simulink model "NavFilterTestHarness24"  (R2016b)
settings: Solver=FixedStepDiscrete  StartTime=startTime  StopTime=endTime  FixedStep=0.001  RelTol=1e-3  EnableMultiTasking=on
undefined symbols (not defined in the file): accel, ADSframe, ADStime, alignTime, angRate, ATTframe, CourseDeg, EAS2TAS, GndSpd, GPSframe, GPStime, Hgt, IMUframe, IMUtime, LatDeg, LngDeg, MagBiasX, MagBiasY, MagBiasZ, MAGframe, MAGtime, MagX, MagY, MagZ, msecHgtDelay, msecMagDelay, msecPosDelay, msecTasDelay, msecVelDelay, Pitch, Roll, Veas, VelD, Yaw
libraries: simulink x9, simulink_need_slupdate x2
(part 4 of 5)

== matlab function NavFilterTestHarness24/InertialNavFilter/Fuse True Airspeed Measurements ==
  data: states input; P input; FuseData input; VtasMea input; nextStates output; nextP output; innovation output; StatesAtMeasTime input; varInnov output; useAirspeed input
%#codegen
function [...
    nextStates, ... % state vector after fusion of measurements
    nextP, ... % state covariance matrix after fusion of corrections
    innovation, ... % True airspeed innovations (m/s)
    varInnov] ... % True airspeed innovation variance (m/s)^2
    = FuseAirspeed( ...
    states, ... % predicted states from the INS (q0, ... , q3, VelN,E,D, PosN,E,D, WindN,E, P0, camera roll pitch yaw misalignment)
    P, ... % predicted covariance
    FuseData, ... % Boolean to initiate fusion of airspeed measurements
    VtasMea, ... % true airspeed measurement (m/s)
    StatesAtMeasTime, ... % states at time of airspeed measurement
    useAirspeed) % Boolean to indicate that a airspeed sensor is being used

% define arrays used to calculate intermediate result in covariance
% update
KH  = single(zeros(24,24));
KHP = single(zeros(24,24));

% initialise innovation
innovation = single(0);

% initialise innovation variance vector (for data analysis only)
varInnov = single(0);

% Airspeed measurement error variance (m/s)^2.
R_TAS = single(2.0);

% Copy required states to local variable names
vn = single(StatesAtMeasTime(5));
ve = single(StatesAtMeasTime(6));
vd = single(StatesAtMeasTime(7));
vwn = single(StatesAtMeasTime(17));
vwe = single(StatesAtMeasTime(18));

% Calculate the airspeed prediction
VtasPred = sqrt((ve - vwe)^2 + (vn - vwn)^2 + vd^2);
% Need to check that it is flying before fusing airspeed data due to
if (useAirspeed && FuseData && (VtasPred > 1.0) && VtasMea > 8.0)
    % Sequential fusion of XYZ components
    
    % Calculate observation jacobians
    SH_TAS = single(zeros(3,1));
    SH_TAS(1) = 1/VtasPred;
    SH_TAS(2) = (SH_TAS(1)*(2*ve - 2*vwe))/2;
    SH_TAS(3) = (SH_TAS(1)*(2*vn - 2*vwn))/2;
    
    H_TAS = single(zeros(1,24));
    H_TAS(1,5) = SH_TAS(3);
    H_TAS(1,6) = SH_TAS(2);
    H_TAS(1,7) = vd*SH_TAS(1);
    H_TAS(1,17) = -SH_TAS(3);
    H_TAS(1,18) = -SH_TAS(2);
    
    SK_TAS = 1/(R_TAS + SH_TAS(3)*(P(5,5)*SH_TAS(3) + P(6,5)*SH_TAS(2) - P(17,5)*SH_TAS(3) - P(18,5)*SH_TAS(2) + P(7,5)*vd*SH_TAS(1)) + SH_TAS(2)*(P(5,6)*SH_TAS(3) + P(6,6)*SH_TAS(2) - P(17,6)*SH_TAS(3) - P(18,6)*SH_TAS(2) + P(7,6)*vd*SH_TAS(1)) - SH_TAS(3)*(P(5,17)*SH_TAS(3) + P(6,17)*SH_TAS(2) - P(17,17)*SH_TAS(3) - P(18,17)*SH_TAS(2) + P(7,17)*vd*SH_TAS(1)) - SH_TAS(2)*(P(5,18)*SH_TAS(3) + P(6,18)*SH_TAS(2) - P(17,18)*SH_TAS(3) - P(18,18)*SH_TAS(2) + P(7,18)*vd*SH_TAS(1)) + vd*SH_TAS(1)*(P(5,7)*SH_TAS(3) + P(6,7)*SH_TAS(2) - P(17,7)*SH_TAS(3) - P(18,7)*SH_TAS(2) + P(7,7)*vd*SH_TAS(1)));
    
    K_TAS = single(zeros(24,1));
    K_TAS(1,1) = SK_TAS*(P(1,5)*SH_TAS(3) - P(1,17)*SH_TAS(3) + P(1,6)*SH_TAS(2) - P(1,18)*SH_TAS(2) + P(1,7)*vd*SH_TAS(1));
    K_TAS(2,1) = SK_TAS*(P(2,5)*SH_TAS(3) - P(2,17)*SH_TAS(3) + P(2,6)*SH_TAS(2) - P(2,18)*SH_TAS(2) + P(2,7)*vd*SH_TAS(1));
    K_TAS(3,1) = SK_TAS*(P(3,5)*SH_TAS(3) - P(3,17)*SH_TAS(3) + P(3,6)*SH_TAS(2) - P(3,18)*SH_TAS(2) + P(3,7)*vd*SH_TAS(1));
    K_TAS(4,1) = SK_TAS*(P(4,5)*SH_TAS(3) - P(4,17)*SH_TAS(3) + P(4,6)*SH_TAS(2) - P(4,18)*SH_TAS(2) + P(4,7)*vd*SH_TAS(1));
    K_TAS(5,1) = SK_TAS*(P(5,5)*SH_TAS(3) - P(5,17)*SH_TAS(3) + P(5,6)*SH_TAS(2) - P(5,18)*SH_TAS(2) + P(5,7)*vd*SH_TAS(1));
    K_TAS(6,1) = SK_TAS*(P(6,5)*SH_TAS(3) - P(6,17)*SH_TAS(3) + P(6,6)*SH_TAS(2) - P(6,18)*SH_TAS(2) + P(6,7)*vd*SH_TAS(1));
    K_TAS(7,1) = SK_TAS*(P(7,5)*SH_TAS(3) - P(7,17)*SH_TAS(3) + P(7,6)*SH_TAS(2) - P(7,18)*SH_TAS(2) + P(7,7)*vd*SH_TAS(1));
    K_TAS(8,1) = SK_TAS*(P(8,5)*SH_TAS(3) - P(8,17)*SH_TAS(3) + P(8,6)*SH_TAS(2) - P(8,18)*SH_TAS(2) + P(8,7)*vd*SH_TAS(1));
    K_TAS(9,1) = SK_TAS*(P(9,5)*SH_TAS(3) - P(9,17)*SH_TAS(3) + P(9,6)*SH_TAS(2) - P(9,18)*SH_TAS(2) + P(9,7)*vd*SH_TAS(1));
    K_TAS(10,1) = SK_TAS*(P(10,5)*SH_TAS(3) - P(10,17)*SH_TAS(3) + P(10,6)*SH_TAS(2) - P(10,18)*SH_TAS(2) + P(10,7)*vd*SH_TAS(1));
    K_TAS(11,1) = SK_TAS*(P(11,5)*SH_TAS(3) - P(11,17)*SH_TAS(3) + P(11,6)*SH_TAS(2) - P(11,18)*SH_TAS(2) + P(11,7)*vd*SH_TAS(1));
    K_TAS(12,1) = SK_TAS*(P(12,5)*SH_TAS(3) - P(12,17)*SH_TAS(3) + P(12,6)*SH_TAS(2) - P(12,18)*SH_TAS(2) + P(12,7)*vd*SH_TAS(1));
    K_TAS(13,1) = SK_TAS*(P(13,5)*SH_TAS(3) - P(13,17)*SH_TAS(3) + P(13,6)*SH_TAS(2) - P(13,18)*SH_TAS(2) + P(13,7)*vd*SH_TAS(1));
    K_TAS(14,1) = SK_TAS*(P(14,5)*SH_TAS(3) - P(14,17)*SH_TAS(3) + P(14,6)*SH_TAS(2) - P(14,18)*SH_TAS(2) + P(14,7)*vd*SH_TAS(1));
    K_TAS(15,1) = SK_TAS*(P(15,5)*SH_TAS(3) - P(15,17)*SH_TAS(3) + P(15,6)*SH_TAS(2) - P(15,18)*SH_TAS(2) + P(15,7)*vd*SH_TAS(1));
    K_TAS(16,1) = SK_TAS*(P(16,5)*SH_TAS(3) - P(16,17)*SH_TAS(3) + P(16,6)*SH_TAS(2) - P(16,18)*SH_TAS(2) + P(16,7)*vd*SH_TAS(1));
    K_TAS(17,1) = SK_TAS*(P(17,5)*SH_TAS(3) - P(17,17)*SH_TAS(3) + P(17,6)*SH_TAS(2) - P(17,18)*SH_TAS(2) + P(17,7)*vd*SH_TAS(1));
    K_TAS(18,1) = SK_TAS*(P(18,5)*SH_TAS(3) - P(18,17)*SH_TAS(3) + P(18,6)*SH_TAS(2) - P(18,18)*SH_TAS(2) + P(18,7)*vd*SH_TAS(1));
    K_TAS(19,1) = SK_TAS*(P(19,5)*SH_TAS(3) - P(19,17)*SH_TAS(3) + P(19,6)*SH_TAS(2) - P(19,18)*SH_TAS(2) + P(19,7)*vd*SH_TAS(1));
    K_TAS(20,1) = SK_TAS*(P(20,5)*SH_TAS(3) - P(20,17)*SH_TAS(3) + P(20,6)*SH_TAS(2) - P(20,18)*SH_TAS(2) + P(20,7)*vd*SH_TAS(1));
    K_TAS(21,1) = SK_TAS*(P(21,5)*SH_TAS(3) - P(21,17)*SH_TAS(3) + P(21,6)*SH_TAS(2) - P(21,18)*SH_TAS(2) + P(21,7)*vd*SH_TAS(1));
    K_TAS(22,1) = SK_TAS*(P(22,5)*SH_TAS(3) - P(22,17)*SH_TAS(3) + P(22,6)*SH_TAS(2) - P(22,18)*SH_TAS(2) + P(22,7)*vd*SH_TAS(1));
    K_TAS(23,1) = SK_TAS*(P(23,5)*SH_TAS(3) - P(23,17)*SH_TAS(3) + P(23,6)*SH_TAS(2) - P(23,18)*SH_TAS(2) + P(23,7)*vd*SH_TAS(1));
    K_TAS(24,1) = SK_TAS*(P(24,5)*SH_TAS(3) - P(24,17)*SH_TAS(3) + P(24,6)*SH_TAS(2) - P(24,18)*SH_TAS(2) + P(24,7)*vd*SH_TAS(1));
    
    % calculate the innovation variance (for data logging only)
    varInnov = 1/SK_TAS;
    
    % correct the states
    innovation = VtasPred - VtasMea;
    % Check the innovation for consistencey and don't fuse if > 5 Sigma
    if (SK_TAS * innovation^2) < 25.0
        xk = K_TAS * innovation;
        states = states - xk;
        % Normalise the quaternion states
        quatMag = sqrt(states(1)^2 + states(2)^2 + states(3)^2 + states(4)^2);
        if (quatMag > 1e-12)
            states(1:4) = states(1:4) / quatMag;
        end
        % correct the covariance P = (I - K*H)*P
        % take advantage of the empty columns in H_TAS to reduce the
        % number of operations
        for i = 1:24
            for j = 5:7
                KH(i,j) = K_TAS(i)*H_TAS(j);
            end
            for j = 17:18
                KH(i,j) = K_TAS(i)*H_TAS(j);
            end
        end
        for i = 1:24
            for j = 1:24
                for k = 5:7
                    KHP(i,j) = KHP(i,j) + KH(i,k)*P(k,j);
                end
                for k = 17:18
                    KHP(i,j) = KHP(i,j) + KH(i,k)*P(k,j);
                end
            end
        end
        P = P - KHP;
    end
end

% Set output for states and covariance
nextP = P;
nextStates   = states;

end

== matlab function NavFilterTestHarness24/InertialNavFilter/Recall States2 ==
  data: fuseData output; statesStore input; msecStore input; msecDelay input; statesOut output; states input; time input; newDataArrived input
%#codegen
function [fuseData,statesOut]    = RecallStates2(statesStore,msecStore,msecDelay,states,time,newDataArrived)
persistent statesForFusion;
if isempty(statesForFusion)
    statesForFusion = single(zeros(24,1));
end
bestTimeDelta = int32(msecDelay);
bestStoreIndex = 1;
if newDataArrived
    for storeIndex=1:50
        timeDelta = (int32(time*1000) - int32(msecDelay)) - int32(msecStore(storeIndex));
        if (timeDelta < 0)
            timeDelta = -timeDelta;
        end
        if (timeDelta < bestTimeDelta)
            bestStoreIndex = storeIndex;
            bestTimeDelta = timeDelta;
        end
    end
    if (bestTimeDelta < msecDelay) % only output stored state if time accuracy better than just outputtting current states
        for i=1:24
            statesForFusion(i) = statesStore(i,bestStoreIndex);
        end
    else % otherwise output current state
        for i=1:24
            statesForFusion(i) = states(i);
        end
    end
end
statesOut = statesForFusion;
fuseData = newDataArrived;
end

== matlab function NavFilterTestHarness24/InertialNavFilter/Calc Initial Parameters/Embedded MATLAB Function ==
  data: earthRateNED output; covariance output; latDeg input
function [earthRateNED, covariance] = calculateInitialData(latDeg)
%#codegen

% degrees to to radians conversion
deg2rad = single(pi/180);

% Define the initial Euler angle covariance (Phi, Theta, Psi)
InitialEulerCovariance  = single([(1.0*pi/180); (1.0*pi/180); (10.0*pi/180)].^2);

% Define the transformation vector from a 321 sequence Euler rotation vector to a q0,...,q3 quaternion vector
% linearised around a level orientation (roll,pitch = 0,0)
J_eul2quat = ...
    single([[ 0.0, 0.0, 0.0]; ...
    [ 0.5, 0.0, 0.0]; ...
    [ 0.0, 0.5, 0.0]; ...
    [ 0.0, 0.0, 0.5]]);

% Form the covariance matrix for the intial Euler angle coordinates
angleCov = diag(InitialEulerCovariance);

% Transform the Euler angle covariances into the equivalent quaternion covariances
quatCov = J_eul2quat*angleCov*transpose(J_eul2quat);

% define the state covariances with the exception of the quaternion covariances
Sigma_vel_NE = single(0.7); % 1 sigma uncertainty in horizontal velocity components
Sigma_vel_D  = single(0.7); % 1 sigma uncertainty in vertical velocity
Sigma_pos_NE = single(15); % 1 sigma uncertainty in horizontal position components
Sigma_pos_D  = single(5.0); % 1 sigma uncertainty in vertical position
Sigma_dAng   = single(1/10*pi/180*0.02); % 1 Sigma uncertainty in delta angle bias
Sigma_dVel   = single(0.1*0.02); % 1 Sigma uncertainty in delta velocity bias
Sigma_wind   = single(8);
Sigma_MagNED = single(20);
Sigma_MagXYZ = single(20);
covariance   = single(diag([0;0;0;0;Sigma_vel_NE*[1;1];Sigma_vel_D;Sigma_pos_NE*[1;1];Sigma_pos_D;Sigma_dAng*[1;1;1];Sigma_dVel*[1;1;1];Sigma_wind*[1;1];Sigma_MagNED*[1;1;1];Sigma_MagXYZ*[1;1;1]].^2));

% Add the quaternion covariances
covariance(1:4,1:4) = quatCov;

%Define Earth rotation vector in the NED navigation frame
earthRateECEF = single([0; 0; 7.2921e-005]);
earthRateNED  = ...
    single([cos(latDeg*deg2rad)*earthRateECEF(3); ...
    0; ...
    -sin(latDeg*deg2rad)*earthRateECEF(3)]);

== matlab function NavFilterTestHarness24/InertialNavFilter/Recall States3 ==
  data: fuseData output; statesStore input; msecStore input; msecDelay input; statesOut output; states input; time input; newDataArrived input
%#codegen
function [fuseData,statesOut]    = RecallStates3(statesStore,msecStore,msecDelay,states,time,newDataArrived)
persistent statesForFusion;
if isempty(statesForFusion)
    statesForFusion = single(zeros(24,1));
end
bestTimeDelta = int32(msecDelay);
bestStoreIndex = 1;
if newDataArrived
    for storeIndex=1:50
        timeDelta = (int32(time*1000) - int32(msecDelay)) - int32(msecStore(storeIndex));
        if (timeDelta < 0)
            timeDelta = -timeDelta;
        end
        if (timeDelta < bestTimeDelta)
            bestStoreIndex = storeIndex;
            bestTimeDelta = timeDelta;
        end
    end
    if (bestTimeDelta < msecDelay) % only output stored state if time accuracy better than just outputtting current states
        for i=1:24
            statesForFusion(i) = statesStore(i,bestStoreIndex);
        end
    else % otherwise output current state
        for i=1:24
            statesForFusion(i) = states(i);
        end
    end
end
statesOut = statesForFusion;
fuseData = newDataArrived;
end

== matlab function NavFilterTestHarness24/InertialNavFilter/Recall States4 ==
  data: fuseData output; statesStore input; msecStore input; msecDelay input; statesOut output; states input; time input; newDataArrived input
%#codegen
function [fuseData,statesOut]    = RecallStates4(statesStore,msecStore,msecDelay,states,time,newDataArrived)
persistent statesForFusion;
if isempty(statesForFusion)
    statesForFusion = single(zeros(24,1));
end
bestTimeDelta = int32(msecDelay);
bestStoreIndex = 1;
if newDataArrived
    for storeIndex=1:50
        timeDelta = (int32(time*1000) - int32(msecDelay)) - int32(msecStore(storeIndex));
        if (timeDelta < 0)
            timeDelta = -timeDelta;
        end
        if (timeDelta < bestTimeDelta)
            bestStoreIndex = storeIndex;
            bestTimeDelta = timeDelta;
        end
    end
    if (bestTimeDelta < msecDelay) % only output stored state if time accuracy better than just outputtting current states
        for i=1:24
            statesForFusion(i) = statesStore(i,bestStoreIndex);
        end
    else % otherwise output current state
        for i=1:24
            statesForFusion(i) = states(i);
        end
    end
end
statesOut = statesForFusion;
fuseData = newDataArrived;
end

== matlab function NavFilterTestHarness24/InertialNavFilter/Fuse Magnetometer Measurements ==
  data: states input; P input; FuseData input; MagData input; StatesAtMeasTime input; nextStates output; nextP output; innovation output; varInnov output; useCompass input
%#codegen
function [...
    nextStates, ... % state vector after fusion of measurements
    nextP, ... % state covariance matrix after fusion of corrections
    innovation, ... % Magnetometer innovations - milligauss
    varInnov] ... % Innovation variances - millgauss^2
    = FuseMagnetometer( ...
    states, ... % predicted states
    P, ... % predicted covariance
    FuseData, ... % Boolean to initiate fusion of magnetometer measurements
    MagData, ... % Magnetic flux measurements (milliGauss)
    StatesAtMeasTime, ... % states at time of airspeed measurement
    useCompass) % Boolean to indicate that a Magnetometer is being used

persistent q0 q1 q2 q3 magN magE magD;
if isempty(q0)
    q0 = single(1);
end
if isempty(q1)
    q1 = single(0);
end
if isempty(q2)
    q2 = single(0);
end
if isempty(q3)
    q3 = single(0);
end
if isempty(magN)
    magN = single(0);
end
if isempty(magE)
    magE = single(0);
end
if isempty(magD)
    magD = single(0);
end
persistent obsIndex
if isempty(obsIndex)
    obsIndex = 1;
end
persistent SH_MAG
if isempty(SH_MAG)
    SH_MAG = single(zeros(1,9));
end
persistent Tnb
if isempty(Tnb)
    Tnb = single(eye(3,3));
end
persistent MagPred
if isempty(MagPred)
    MagPred = single(zeros(3,1));
end

% declare arrays used to calculate intermediate result in covariance
% and state update
K_MAG = single(zeros(24,1));
H_MAG = single(zeros(1,24));
KH    = single(zeros(24,24));
KHP = single(zeros(24,24));
% define magnetometer measurement error variance (milligauss).
R_MAG = single(50^2);
% declare innovation variances
varInnov = single(zeros(3,1));
% declare innovation vector
innovation = single(zeros(1,3));
% Perform sequential fusion of Magnetometer measurements.
% This assumes that the errors in the dfferent componenets are
% uncorrelated which is not true, however in the absence of covariance
% data fit is the only assumption we can make
% so we might as well take advantage of the computational efficiencies
% associated with sequential fusion
if (useCompass && FuseData) || (useCompass && (obsIndex == 2 || obsIndex == 3))
    % Sequential fusion of XYZ components to spread processing load across
    % three prediction time steps.
    % Calculate observation jacobians and Kalman gains
    if FuseData
        % Copy required states to local variable names
        q0 = StatesAtMeasTime(1);
        q1 = StatesAtMeasTime(2);
        q2 = StatesAtMeasTime(3);
        q3 = StatesAtMeasTime(4);
        magN = StatesAtMeasTime(19);
        magE = StatesAtMeasTime(20);
        magD = StatesAtMeasTime(21);
        % rotate predicted earth components into body axes and calculate
        % predicted measurments
        Tnb = single([q0^2 + q1^2 - q2^2 - q3^2, 2*(q1*q2 + q0*q3) , 2*(q1*q3-q0*q2) ;...
            2*(q1*q2 - q0*q3), q0^2 - q1^2 + q2^2 - q3^2, 2*(q2*q3 + q0*q1);...
            2*(q1*q3 + q0*q2) , 2*(q2*q3 - q0*q1) , q0^2 - q1^2 - q2^2 + q3^2]);
        MagPred = Tnb*StatesAtMeasTime(19:21) + StatesAtMeasTime(22:24);
        % Calculate observation jacobian common terms
        SH_MAG(1) = 2*magD*q3 + 2*magE*q2 + 2*magN*q1;
        SH_MAG(2) = 2*magD*q0 - 2*magE*q1 + 2*magN*q2;
        SH_MAG(3) = 2*magD*q1 + 2*magE*q0 - 2*magN*q3;
        SH_MAG(4) = q3^2;
        SH_MAG(5) = q2^2;
        SH_MAG(6) = q1^2;
        SH_MAG(7) = q0^2;
        SH_MAG(8) = 2*magN*q0;
        SH_MAG(9) = 2*magE*q3;
        % calculate observation jacobian
        H_MAG(1,1) = SH_MAG(8) + SH_MAG(9) - 2*magD*q2;
        H_MAG(1,2) = SH_MAG(1);
        H_MAG(1,3) = 2*magE*q1 - 2*magD*q0 - 2*magN*q2;
        H_MAG(1,4) = SH_MAG(3);
        H_MAG(1,19) = SH_MAG(6) - SH_MAG(5) - SH_MAG(4) + SH_MAG(7);
        H_MAG(1,20) = 2*q0*q3 + 2*q1*q2;
        H_MAG(1,21) = 2*q1*q3 - 2*q0*q2;
        H_MAG(1,22) = 1;
        % calculate Kalman gain
        SK_MX = single(zeros(6,1));
        SK_MX(1) = 1/(P(22,22) + R_MAG + P(2,22)*SH_MAG(1) + P(4,22)*SH_MAG(3) - P(19,22)*(SH_MAG(4) + SH_MAG(5) - SH_MAG(6) - SH_MAG(7)) - (2*magD*q0 - 2*magE*q1 + 2*magN*q2)*(P(22,3) + P(2,3)*SH_MAG(1) + P(4,3)*SH_MAG(3) - P(19,3)*(SH_MAG(4) + SH_MAG(5) - SH_MAG(6) - SH_MAG(7)) + P(20,3)*(2*q0*q3 + 2*q1*q2) - P(21,3)*(2*q0*q2 - 2*q1*q3) - P(3,3)*(2*magD*q0 - 2*magE*q1 + 2*magN*q2) + P(1,3)*(SH_MAG(8) + SH_MAG(9) - 2*magD*q2)) + (SH_MAG(8) + SH_MAG(9) - 2*magD*q2)*(P(22,1) + P(2,1)*SH_MAG(1) + P(4,1)*SH_MAG(3) - P(19,1)*(SH_MAG(4) + SH_MAG(5) - SH_MAG(6) - SH_MAG(7)) + P(20,1)*(2*q0*q3 + 2*q1*q2) - P(21,1)*(2*q0*q2 - 2*q1*q3) - P(3,1)*(2*magD*q0 - 2*magE*q1 + 2*magN*q2) + P(1,1)*(SH_MAG(8) + SH_MAG(9) - 2*magD*q2)) + SH_MAG(1)*(P(22,2) + P(2,2)*SH_MAG(1) + P(4,2)*SH_MAG(3) - P(19,2)*(SH_MAG(4) + SH_MAG(5) - SH_MAG(6) - SH_MAG(7)) + P(20,2)*(2*q0*q3 + 2*q1*q2) - P(21,2)*(2*q0*q2 - 2*q1*q3) - P(3,2)*(2*magD*q0 - 2*magE*q1 + 2*magN*q2) + P(1,2)*(SH_MAG(8) + SH_MAG(9) - 2*magD*q2)) + SH_MAG(3)*(P(22,4) + P(2,4)*SH_MAG(1) + P(4,4)*SH_MAG(3) - P(19,4)*(SH_MAG(4) + SH_MAG(5) - SH_MAG(6) - SH_MAG(7)) + P(20,4)*(2*q0*q3 + 2*q1*q2) - P(21,4)*(2*q0*q2 - 2*q1*q3) - P(3,4)*(2*magD*q0 - 2*magE*q1 + 2*magN*q2) + P(1,4)*(SH_MAG(8) + SH_MAG(9) - 2*magD*q2)) - (SH_MAG(4) + SH_MAG(5) - SH_MAG(6) - SH_MAG(7))*(P(22,19) + P(2,19)*SH_MAG(1) + P(4,19)*SH_MAG(3) - P(19,19)*(SH_MAG(4) + SH_MAG(5) - SH_MAG(6) - SH_MAG(7)) + P(20,19)*(2*q0*q3 + 2*q1*q2) - P(21,19)*(2*q0*q2 - 2*q1*q3) - P(3,19)*(2*magD*q0 - 2*magE*q1 + 2*magN*q2) + P(1,19)*(SH_MAG(8) + SH_MAG(9) - 2*magD*q2)) + P(20,22)*(2*q0*q3 + 2*q1*q2) - P(21,22)*(2*q0*q2 - 2*q1*q3) - P(3,22)*(2*magD*q0 - 2*magE*q1 + 2*magN*q2) + (2*q0*q3 + 2*q1*q2)*(P(22,20) + P(2,20)*SH_MAG(1) + P(4,20)*SH_MAG(3) - P(19,20)*(SH_MAG(4) + SH_MAG(5) - SH_MAG(6) - SH_MAG(7)) + P(20,20)*(2*q0*q3 + 2*q1*q2) - P(21,20)*(2*q0*q2 - 2*q1*q3) - P(3,20)*(2*magD*q0 - 2*magE*q1 + 2*magN*q2) + P(1,20)*(SH_MAG(8) + SH_MAG(9) - 2*magD*q2)) - (2*q0*q2 - 2*q1*q3)*(P(22,21) + P(2,21)*SH_MAG(1) + P(4,21)*SH_MAG(3) - P(19,21)*(SH_MAG(4) + SH_MAG(5) - SH_MAG(6) - SH_MAG(7)) + P(20,21)*(2*q0*q3 + 2*q1*q2) - P(21,21)*(2*q0*q2 - 2*q1*q3) - P(3,21)*(2*magD*q0 - 2*magE*q1 + 2*magN*q2) + P(1,21)*(SH_MAG(8) + SH_MAG(9) - 2*magD*q2)) + P(1,22)*(SH_MAG(8) + SH_MAG(9) - 2*magD*q2));
        SK_MX(2) = SH_MAG(4) + SH_MAG(5) - SH_MAG(6) - SH_MAG(7);
        SK_MX(3) = 2*magD*q0 - 2*magE*q1 + 2*magN*q2;
        SK_MX(4) = SH_MAG(8) + SH_MAG(9) - 2*magD*q2;
        SK_MX(5) = 2*q0*q2 - 2*q1*q3;
        SK_MX(6) = 2*q0*q3 + 2*q1*q2;
        K_MAG(1,1) = SK_MX(1)*(P(1,22) + P(1,2)*SH_MAG(1) + P(1,4)*SH_MAG(3) + P(1,1)*SK_MX(4) - P(1,3)*SK_MX(3) - P(1,19)*SK_MX(2) + P(1,20)*SK_MX(6) - P(1,21)*SK_MX(5));
        K_MAG(2,1) = SK_MX(1)*(P(2,22) + P(2,2)*SH_MAG(1) + P(2,4)*SH_MAG(3) + P(2,1)*SK_MX(4) - P(2,3)*SK_MX(3) - P(2,19)*SK_MX(2) + P(2,20)*SK_MX(6) - P(2,21)*SK_MX(5));
        K_MAG(3,1) = SK_MX(1)*(P(3,22) + P(3,2)*SH_MAG(1) + P(3,4)*SH_MAG(3) + P(3,1)*SK_MX(4) - P(3,3)*SK_MX(3) - P(3,19)*SK_MX(2) + P(3,20)*SK_MX(6) - P(3,21)*SK_MX(5));
        K_MAG(4,1) = SK_MX(1)*(P(4,22) + P(4,2)*SH_MAG(1) + P(4,4)*SH_MAG(3) + P(4,1)*SK_MX(4) - P(4,3)*SK_MX(3) - P(4,19)*SK_MX(2) + P(4,20)*SK_MX(6) - P(4,21)*SK_MX(5));
        K_MAG(5,1) = SK_MX(1)*(P(5,22) + P(5,2)*SH_MAG(1) + P(5,4)*SH_MAG(3) + P(5,1)*SK_MX(4) - P(5,3)*SK_MX(3) - P(5,19)*SK_MX(2) + P(5,20)*SK_MX(6) - P(5,21)*SK_MX(5));
        K_MAG(6,1) = SK_MX(1)*(P(6,22) + P(6,2)*SH_MAG(1) + P(6,4)*SH_MAG(3) + P(6,1)*SK_MX(4) - P(6,3)*SK_MX(3) - P(6,19)*SK_MX(2) + P(6,20)*SK_MX(6) - P(6,21)*SK_MX(5));
        K_MAG(7,1) = SK_MX(1)*(P(7,22) + P(7,2)*SH_MAG(1) + P(7,4)*SH_MAG(3) + P(7,1)*SK_MX(4) - P(7,3)*SK_MX(3) - P(7,19)*SK_MX(2) + P(7,20)*SK_MX(6) - P(7,21)*SK_MX(5));
        K_MAG(8,1) = SK_MX(1)*(P(8,22) + P(8,2)*SH_MAG(1) + P(8,4)*SH_MAG(3) + P(8,1)*SK_MX(4) - P(8,3)*SK_MX(3) - P(8,19)*SK_MX(2) + P(8,20)*SK_MX(6) - P(8,21)*SK_MX(5));
        K_MAG(9,1) = SK_MX(1)*(P(9,22) + P(9,2)*SH_MAG(1) + P(9,4)*SH_MAG(3) + P(9,1)*SK_MX(4) - P(9,3)*SK_MX(3) - P(9,19)*SK_MX(2) + P(9,20)*SK_MX(6) - P(9,21)*SK_MX(5));
        K_MAG(10,1) = SK_MX(1)*(P(10,22) + P(10,2)*SH_MAG(1) + P(10,4)*SH_MAG(3) + P(10,1)*SK_MX(4) - P(10,3)*SK_MX(3) - P(10,19)*SK_MX(2) + P(10,20)*SK_MX(6) - P(10,21)*SK_MX(5));
        K_MAG(11,1) = SK_MX(1)*(P(11,22) + P(11,2)*SH_MAG(1) + P(11,4)*SH_MAG(3) + P(11,1)*SK_MX(4) - P(11,3)*SK_MX(3) - P(11,19)*SK_MX(2) + P(11,20)*SK_MX(6) - P(11,21)*SK_MX(5));
        K_MAG(12,1) = SK_MX(1)*(P(12,22) + P(12,2)*SH_MAG(1) + P(12,4)*SH_MAG(3) + P(12,1)*SK_MX(4) - P(12,3)*SK_MX(3) - P(12,19)*SK_MX(2) + P(12,20)*SK_MX(6) - P(12,21)*SK_MX(5));
        K_MAG(13,1) = SK_MX(1)*(P(13,22) + P(13,2)*SH_MAG(1) + P(13,4)*SH_MAG(3) + P(13,1)*SK_MX(4) - P(13,3)*SK_MX(3) - P(13,19)*SK_MX(2) + P(13,20)*SK_MX(6) - P(13,21)*SK_MX(5));
        K_MAG(14,1) = SK_MX(1)*(P(14,22) + P(14,2)*SH_MAG(1) + P(14,4)*SH_MAG(3) + P(14,1)*SK_MX(4) - P(14,3)*SK_MX(3) - P(14,19)*SK_MX(2) + P(14,20)*SK_MX(6) - P(14,21)*SK_MX(5));
        K_MAG(15,1) = SK_MX(1)*(P(15,22) + P(15,2)*SH_MAG(1) + P(15,4)*SH_MAG(3) + P(15,1)*SK_MX(4) - P(15,3)*SK_MX(3) - P(15,19)*SK_MX(2) + P(15,20)*SK_MX(6) - P(15,21)*SK_MX(5));
        K_MAG(16,1) = SK_MX(1)*(P(16,22) + P(16,2)*SH_MAG(1) + P(16,4)*SH_MAG(3) + P(16,1)*SK_MX(4) - P(16,3)*SK_MX(3) - P(16,19)*SK_MX(2) + P(16,20)*SK_MX(6) - P(16,21)*SK_MX(5));
        K_MAG(17,1) = SK_MX(1)*(P(17,22) + P(17,2)*SH_MAG(1) + P(17,4)*SH_MAG(3) + P(17,1)*SK_MX(4) - P(17,3)*SK_MX(3) - P(17,19)*SK_MX(2) + P(17,20)*SK_MX(6) - P(17,21)*SK_MX(5));
        K_MAG(18,1) = SK_MX(1)*(P(18,22) + P(18,2)*SH_MAG(1) + P(18,4)*SH_MAG(3) + P(18,1)*SK_MX(4) - P(18,3)*SK_MX(3) - P(18,19)*SK_MX(2) + P(18,20)*SK_MX(6) - P(18,21)*SK_MX(5));
        K_MAG(19,1) = SK_MX(1)*(P(19,22) + P(19,2)*SH_MAG(1) + P(19,4)*SH_MAG(3) + P(19,1)*SK_MX(4) - P(19,3)*SK_MX(3) - P(19,19)*SK_MX(2) + P(19,20)*SK_MX(6) - P(19,21)*SK_MX(5));
        K_MAG(20,1) = SK_MX(1)*(P(20,22) + P(20,2)*SH_MAG(1) + P(20,4)*SH_MAG(3) + P(20,1)*SK_MX(4) - P(20,3)*SK_MX(3) - P(20,19)*SK_MX(2) + P(20,20)*SK_MX(6) - P(20,21)*SK_MX(5));
        K_MAG(21,1) = SK_MX(1)*(P(21,22) + P(21,2)*SH_MAG(1) + P(21,4)*SH_MAG(3) + P(21,1)*SK_MX(4) - P(21,3)*SK_MX(3) - P(21,19)*SK_MX(2) + P(21,20)*SK_MX(6) - P(21,21)*SK_MX(5));
        K_MAG(22,1) = SK_MX(1)*(P(22,22) + P(22,2)*SH_MAG(1) + P(22,4)*SH_MAG(3) + P(22,1)*SK_MX(4) - P(22,3)*SK_MX(3) - P(22,19)*SK_MX(2) + P(22,20)*SK_MX(6) - P(22,21)*SK_MX(5));
        K_MAG(23,1) = SK_MX(1)*(P(23,22) + P(23,2)*SH_MAG(1) + P(23,4)*SH_MAG(3) + P(23,1)*SK_MX(4) - P(23,3)*SK_MX(3) - P(23,19)*SK_MX(2) + P(23,20)*SK_MX(6) - P(23,21)*SK_MX(5));
        K_MAG(24,1) = SK_MX(1)*(P(24,22) + P(24,2)*SH_MAG(1) + P(24,4)*SH_MAG(3) + P(24,1)*SK_MX(4) - P(24,3)*SK_MX(3) - P(24,19)*SK_MX(2) + P(24,20)*SK_MX(6) - P(24,21)*SK_MX(5));
        varInnov(1) = 1/SK_MX(1);
        % reset the observation index to 1 (we start by fusing the X
        % measurement)
        obsIndex = 1;
    elseif obsIndex == 2 % we are now fusing the Y measurement
        H_MAG(1,1) = SH_MAG(3);
        H_MAG(1,2) = SH_MAG(2);
        H_MAG(1,3) = SH_MAG(1);
        H_MAG(1,4) = 2*magD*q2 - SH_MAG(9) - SH_MAG(8);
        H_MAG(1,19) = 2*q1*q2 - 2*q0*q3;
        H_MAG(1,20) = SH_MAG(5) - SH_MAG(4) - SH_MAG(6) + SH_MAG(7);
        H_MAG(1,21) = 2*q0*q1 + 2*q2*q3;
        H_MAG(1,23) = 1;
        % calculate the Kalman gain
        SK_MY = single(zeros(5,1));
        SK_MY(1) = 1/(P(23,23) + R_MAG + P(1,23)*SH_MAG(3) + P(2,23)*SH_MAG(2) + P(3,23)*SH_MAG(1) - P(20,23)*(SH_MAG(4) - SH_MAG(5) + SH_MAG(6) - SH_MAG(7)) - (2*q0*q3 - 2*q1*q2)*(P(23,19) + P(1,19)*SH_MAG(3) + P(2,19)*SH_MAG(2) + P(3,19)*SH_MAG(1) - P(20,19)*(SH_MAG(4) - SH_MAG(5) + SH_MAG(6) - SH_MAG(7)) - P(19,19)*(2*q0*q3 - 2*q1*q2) + P(21,19)*(2*q0*q1 + 2*q2*q3) - P(4,19)*(SH_MAG(8) + SH_MAG(9) - 2*magD*q2)) + (2*q0*q1 + 2*q2*q3)*(P(23,21) + P(1,21)*SH_MAG(3) + P(2,21)*SH_MAG(2) + P(3,21)*SH_MAG(1) - P(20,21)*(SH_MAG(4) - SH_MAG(5) + SH_MAG(6) - SH_MAG(7)) - P(19,21)*(2*q0*q3 - 2*q1*q2) + P(21,21)*(2*q0*q1 + 2*q2*q3) - P(4,21)*(SH_MAG(8) + SH_MAG(9) - 2*magD*q2)) - (SH_MAG(8) + SH_MAG(9) - 2*magD*q2)*(P(23,4) + P(1,4)*SH_MAG(3) + P(2,4)*SH_MAG(2) + P(3,4)*SH_MAG(1) - P(20,4)*(SH_MAG(4) - SH_MAG(5) + SH_MAG(6) - SH_MAG(7)) - P(19,4)*(2*q0*q3 - 2*q1*q2) + P(21,4)*(2*q0*q1 + 2*q2*q3) - P(4,4)*(SH_MAG(8) + SH_MAG(9) - 2*magD*q2)) - P(19,23)*(2*q0*q3 - 2*q1*q2) + P(21,23)*(2*q0*q1 + 2*q2*q3) + SH_MAG(3)*(P(23,1) + P(1,1)*SH_MAG(3) + P(2,1)*SH_MAG(2) + P(3,1)*SH_MAG(1) - P(20,1)*(SH_MAG(4) - SH_MAG(5) + SH_MAG(6) - SH_MAG(7)) - P(19,1)*(2*q0*q3 - 2*q1*q2) + P(21,1)*(2*q0*q1 + 2*q2*q3) - P(4,1)*(SH_MAG(8) + SH_MAG(9) - 2*magD*q2)) + SH_MAG(2)*(P(23,2) + P(1,2)*SH_MAG(3) + P(2,2)*SH_MAG(2) + P(3,2)*SH_MAG(1) - P(20,2)*(SH_MAG(4) - SH_MAG(5) + SH_MAG(6) - SH_MAG(7)) - P(19,2)*(2*q0*q3 - 2*q1*q2) + P(21,2)*(2*q0*q1 + 2*q2*q3) - P(4,2)*(SH_MAG(8) + SH_MAG(9) - 2*magD*q2)) + SH_MAG(1)*(P(23,3) + P(1,3)*SH_MAG(3) + P(2,3)*SH_MAG(2) + P(3,3)*SH_MAG(1) - P(20,3)*(SH_MAG(4) - SH_MAG(5) + SH_MAG(6) - SH_MAG(7)) - P(19,3)*(2*q0*q3 - 2*q1*q2) + P(21,3)*(2*q0*q1 + 2*q2*q3) - P(4,3)*(SH_MAG(8) + SH_MAG(9) - 2*magD*q2)) - (SH_MAG(4) - SH_MAG(5) + SH_MAG(6) - SH_MAG(7))*(P(23,20) + P(1,20)*SH_MAG(3) + P(2,20)*SH_MAG(2) + P(3,20)*SH_MAG(1) - P(20,20)*(SH_MAG(4) - SH_MAG(5) + SH_MAG(6) - SH_MAG(7)) - P(19,20)*(2*q0*q3 - 2*q1*q2) + P(21,20)*(2*q0*q1 + 2*q2*q3) - P(4,20)*(SH_MAG(8) + SH_MAG(9) - 2*magD*q2)) - P(4,23)*(SH_MAG(8) + SH_MAG(9) - 2*magD*q2));
        SK_MY(2) = SH_MAG(4) - SH_MAG(5) + SH_MAG(6) - SH_MAG(7);
        SK_MY(3) = SH_MAG(8) + SH_MAG(9) - 2*magD*q2;
        SK_MY(4) = 2*q0*q3 - 2*q1*q2;
        SK_MY(5) = 2*q0*q1 + 2*q2*q3;
        K_MAG(1,1) = SK_MY(1)*(P(1,23) + P(1,1)*SH_MAG(3) + P(1,2)*SH_MAG(2) + P(1,3)*SH_MAG(1) - P(1,4)*SK_MY(3) - P(1,20)*SK_MY(2) - P(1,19)*SK_MY(4) + P(1,21)*SK_MY(5));
        K_MAG(2,1) = SK_MY(1)*(P(2,23) + P(2,1)*SH_MAG(3) + P(2,2)*SH_MAG(2) + P(2,3)*SH_MAG(1) - P(2,4)*SK_MY(3) - P(2,20)*SK_MY(2) - P(2,19)*SK_MY(4) + P(2,21)*SK_MY(5));
        K_MAG(3,1) = SK_MY(1)*(P(3,23) + P(3,1)*SH_MAG(3) + P(3,2)*SH_MAG(2) + P(3,3)*SH_MAG(1) - P(3,4)*SK_MY(3) - P(3,20)*SK_MY(2) - P(3,19)*SK_MY(4) + P(3,21)*SK_MY(5));
        K_MAG(4,1) = SK_MY(1)*(P(4,23) + P(4,1)*SH_MAG(3) + P(4,2)*SH_MAG(2) + P(4,3)*SH_MAG(1) - P(4,4)*SK_MY(3) - P(4,20)*SK_MY(2) - P(4,19)*SK_MY(4) + P(4,21)*SK_MY(5));
        K_MAG(5,1) = SK_MY(1)*(P(5,23) + P(5,1)*SH_MAG(3) + P(5,2)*SH_MAG(2) + P(5,3)*SH_MAG(1) - P(5,4)*SK_MY(3) - P(5,20)*SK_MY(2) - P(5,19)*SK_MY(4) + P(5,21)*SK_MY(5));
        K_MAG(6,1) = SK_MY(1)*(P(6,23) + P(6,1)*SH_MAG(3) + P(6,2)*SH_MAG(2) + P(6,3)*SH_MAG(1) - P(6,4)*SK_MY(3) - P(6,20)*SK_MY(2) - P(6,19)*SK_MY(4) + P(6,21)*SK_MY(5));
        K_MAG(7,1) = SK_MY(1)*(P(7,23) + P(7,1)*SH_MAG(3) + P(7,2)*SH_MAG(2) + P(7,3)*SH_MAG(1) - P(7,4)*SK_MY(3) - P(7,20)*SK_MY(2) - P(7,19)*SK_MY(4) + P(7,21)*SK_MY(5));
        K_MAG(8,1) = SK_MY(1)*(P(8,23) + P(8,1)*SH_MAG(3) + P(8,2)*SH_MAG(2) + P(8,3)*SH_MAG(1) - P(8,4)*SK_MY(3) - P(8,20)*SK_MY(2) - P(8,19)*SK_MY(4) + P(8,21)*SK_MY(5));
        K_MAG(9,1) = SK_MY(1)*(P(9,23) + P(9,1)*SH_MAG(3) + P(9,2)*SH_MAG(2) + P(9,3)*SH_MAG(1) - P(9,4)*SK_MY(3) - P(9,20)*SK_MY(2) - P(9,19)*SK_MY(4) + P(9,21)*SK_MY(5));
        K_MAG(10,1) = SK_MY(1)*(P(10,23) + P(10,1)*SH_MAG(3) + P(10,2)*SH_MAG(2) + P(10,3)*SH_MAG(1) - P(10,4)*SK_MY(3) - P(10,20)*SK_MY(2) - P(10,19)*SK_MY(4) + P(10,21)*SK_MY(5));
        K_MAG(11,1) = SK_MY(1)*(P(11,23) + P(11,1)*SH_MAG(3) + P(11,2)*SH_MAG(2) + P(11,3)*SH_MAG(1) - P(11,4)*SK_MY(3) - P(11,20)*SK_MY(2) - P(11,19)*SK_MY(4) + P(11,21)*SK_MY(5));
        K_MAG(12,1) = SK_MY(1)*(P(12,23) + P(12,1)*SH_MAG(3) + P(12,2)*SH_MAG(2) + P(12,3)*SH_MAG(1) - P(12,4)*SK_MY(3) - P(12,20)*SK_MY(2) - P(12,19)*SK_MY(4) + P(12,21)*SK_MY(5));
        K_MAG(13,1) = SK_MY(1)*(P(13,23) + P(13,1)*SH_MAG(3) + P(13,2)*SH_MAG(2) + P(13,3)*SH_MAG(1) - P(13,4)*SK_MY(3) - P(13,20)*SK_MY(2) - P(13,19)*SK_MY(4) + P(13,21)*SK_MY(5));
        K_MAG(14,1) = SK_MY(1)*(P(14,23) + P(14,1)*SH_MAG(3) + P(14,2)*SH_MAG(2) + P(14,3)*SH_MAG(1) - P(14,4)*SK_MY(3) - P(14,20)*SK_MY(2) - P(14,19)*SK_MY(4) + P(14,21)*SK_MY(5));
        K_MAG(15,1) = SK_MY(1)*(P(15,23) + P(15,1)*SH_MAG(3) + P(15,2)*SH_MAG(2) + P(15,3)*SH_MAG(1) - P(15,4)*SK_MY(3) - P(15,20)*SK_MY(2) - P(15,19)*SK_MY(4) + P(15,21)*SK_MY(5));
        K_MAG(16,1) = SK_MY(1)*(P(16,23) + P(16,1)*SH_MAG(3) + P(16,2)*SH_MAG(2) + P(16,3)*SH_MAG(1) - P(16,4)*SK_MY(3) - P(16,20)*SK_MY(2) - P(16,19)*SK_MY(4) + P(16,21)*SK_MY(5));
        K_MAG(17,1) = SK_MY(1)*(P(17,23) + P(17,1)*SH_MAG(3) + P(17,2)*SH_MAG(2) + P(17,3)*SH_MAG(1) - P(17,4)*SK_MY(3) - P(17,20)*SK_MY(2) - P(17,19)*SK_MY(4) + P(17,21)*SK_MY(5));
        K_MAG(18,1) = SK_MY(1)*(P(18,23) + P(18,1)*SH_MAG(3) + P(18,2)*SH_MAG(2) + P(18,3)*SH_MAG(1) - P(18,4)*SK_MY(3) - P(18,20)*SK_MY(2) - P(18,19)*SK_MY(4) + P(18,21)*SK_MY(5));
        K_MAG(19,1) = SK_MY(1)*(P(19,23) + P(19,1)*SH_MAG(3) + P(19,2)*SH_MAG(2) + P(19,3)*SH_MAG(1) - P(19,4)*SK_MY(3) - P(19,20)*SK_MY(2) - P(19,19)*SK_MY(4) + P(19,21)*SK_MY(5));
        K_MAG(20,1) = SK_MY(1)*(P(20,23) + P(20,1)*SH_MAG(3) + P(20,2)*SH_MAG(2) + P(20,3)*SH_MAG(1) - P(20,4)*SK_MY(3) - P(20,20)*SK_MY(2) - P(20,19)*SK_MY(4) + P(20,21)*SK_MY(5));
        K_MAG(21,1) = SK_MY(1)*(P(21,23) + P(21,1)*SH_MAG(3) + P(21,2)*SH_MAG(2) + P(21,3)*SH_MAG(1) - P(21,4)*SK_MY(3) - P(21,20)*SK_MY(2) - P(21,19)*SK_MY(4) + P(21,21)*SK_MY(5));
        K_MAG(22,1) = SK_MY(1)*(P(22,23) + P(22,1)*SH_MAG(3) + P(22,2)*SH_MAG(2) + P(22,3)*SH_MAG(1) - P(22,4)*SK_MY(3) - P(22,20)*SK_MY(2) - P(22,19)*SK_MY(4) + P(22,21)*SK_MY(5));
        K_MAG(23,1) = SK_MY(1)*(P(23,23) + P(23,1)*SH_MAG(3) + P(23,2)*SH_MAG(2) + P(23,3)*SH_MAG(1) - P(23,4)*SK_MY(3) - P(23,20)*SK_MY(2) - P(23,19)*SK_MY(4) + P(23,21)*SK_MY(5));
        K_MAG(24,1) = SK_MY(1)*(P(24,23) + P(24,1)*SH_MAG(3) + P(24,2)*SH_MAG(2) + P(24,3)*SH_MAG(1) - P(24,4)*SK_MY(3) - P(24,20)*SK_MY(2) - P(24,19)*SK_MY(4) + P(24,21)*SK_MY(5));
        varInnov(2) = 1/SK_MY(1);
    elseif obsIndex == 3 % we ar now fusing the Z measurement
        % calculate the observation jacobian
        H_MAG(1,1) = SH_MAG(2);
        H_MAG(1,2) = 2*magN*q3 - 2*magE*q0 - 2*magD*q1;
        H_MAG(1,3) = SH_MAG(8) + SH_MAG(9) - 2*magD*q2;
        H_MAG(1,4) = SH_MAG(1);
        H_MAG(1,19) = 2*q0*q2 + 2*q1*q3;
        H_MAG(1,20) = 2*q2*q3 - 2*q0*q1;
        H_MAG(1,21) = SH_MAG(4) - SH_MAG(5) - SH_MAG(6) + SH_MAG(7);
        H_MAG(1,24) = 1;
        % calculate the Kalman gain
        SK_MZ = single(zeros(6,1));
        SK_MZ(1) = 1/(P(24,24) + R_MAG + P(1,24)*SH_MAG(2) + P(4,24)*SH_MAG(1) + P(21,24)*(SH_MAG(4) - SH_MAG(5) - SH_MAG(6) + SH_MAG(7)) - (2*magD*q1 + 2*magE*q0 - 2*magN*q3)*(P(24,2) + P(1,2)*SH_MAG(2) + P(4,2)*SH_MAG(1) + P(21,2)*(SH_MAG(4) - SH_MAG(5) - SH_MAG(6) + SH_MAG(7)) + P(19,2)*(2*q0*q2 + 2*q1*q3) - P(20,2)*(2*q0*q1 - 2*q2*q3) - P(2,2)*(2*magD*q1 + 2*magE*q0 - 2*magN*q3) + P(3,2)*(SH_MAG(8) + SH_MAG(9) - 2*magD*q2)) + (SH_MAG(8) + SH_MAG(9) - 2*magD*q2)*(P(24,3) + P(1,3)*SH_MAG(2) + P(4,3)*SH_MAG(1) + P(21,3)*(SH_MAG(4) - SH_MAG(5) - SH_MAG(6) + SH_MAG(7)) + P(19,3)*(2*q0*q2 + 2*q1*q3) - P(20,3)*(2*q0*q1 - 2*q2*q3) - P(2,3)*(2*magD*q1 + 2*magE*q0 - 2*magN*q3) + P(3,3)*(SH_MAG(8) + SH_MAG(9) - 2*magD*q2)) + SH_MAG(2)*(P(24,1) + P(1,1)*SH_MAG(2) + P(4,1)*SH_MAG(1) + P(21,1)*(SH_MAG(4) - SH_MAG(5) - SH_MAG(6) + SH_MAG(7)) + P(19,1)*(2*q0*q2 + 2*q1*q3) - P(20,1)*(2*q0*q1 - 2*q2*q3) - P(2,1)*(2*magD*q1 + 2*magE*q0 - 2*magN*q3) + P(3,1)*(SH_MAG(8) + SH_MAG(9) - 2*magD*q2)) + SH_MAG(1)*(P(24,4) + P(1,4)*SH_MAG(2) + P(4,4)*SH_MAG(1) + P(21,4)*(SH_MAG(4) - SH_MAG(5) - SH_MAG(6) + SH_MAG(7)) + P(19,4)*(2*q0*q2 + 2*q1*q3) - P(20,4)*(2*q0*q1 - 2*q2*q3) - P(2,4)*(2*magD*q1 + 2*magE*q0 - 2*magN*q3) + P(3,4)*(SH_MAG(8) + SH_MAG(9) - 2*magD*q2)) + (SH_MAG(4) - SH_MAG(5) - SH_MAG(6) + SH_MAG(7))*(P(24,21) + P(1,21)*SH_MAG(2) + P(4,21)*SH_MAG(1) + P(21,21)*(SH_MAG(4) - SH_MAG(5) - SH_MAG(6) + SH_MAG(7)) + P(19,21)*(2*q0*q2 + 2*q1*q3) - P(20,21)*(2*q0*q1 - 2*q2*q3) - P(2,21)*(2*magD*q1 + 2*magE*q0 - 2*magN*q3) + P(3,21)*(SH_MAG(8) + SH_MAG(9) - 2*magD*q2)) + P(19,24)*(2*q0*q2 + 2*q1*q3) - P(20,24)*(2*q0*q1 - 2*q2*q3) - P(2,24)*(2*magD*q1 + 2*magE*q0 - 2*magN*q3) + (2*q0*q2 + 2*q1*q3)*(P(24,19) + P(1,19)*SH_MAG(2) + P(4,19)*SH_MAG(1) + P(21,19)*(SH_MAG(4) - SH_MAG(5) - SH_MAG(6) + SH_MAG(7)) + P(19,19)*(2*q0*q2 + 2*q1*q3) - P(20,19)*(2*q0*q1 - 2*q2*q3) - P(2,19)*(2*magD*q1 + 2*magE*q0 - 2*magN*q3) + P(3,19)*(SH_MAG(8) + SH_MAG(9) - 2*magD*q2)) - (2*q0*q1 - 2*q2*q3)*(P(24,20) + P(1,20)*SH_MAG(2) + P(4,20)*SH_MAG(1) + P(21,20)*(SH_MAG(4) - SH_MAG(5) - SH_MAG(6) + SH_MAG(7)) + P(19,20)*(2*q0*q2 + 2*q1*q3) - P(20,20)*(2*q0*q1 - 2*q2*q3) - P(2,20)*(2*magD*q1 + 2*magE*q0 - 2*magN*q3) + P(3,20)*(SH_MAG(8) + SH_MAG(9) - 2*magD*q2)) + P(3,24)*(SH_MAG(8) + SH_MAG(9) - 2*magD*q2));
        SK_MZ(2) = SH_MAG(4) - SH_MAG(5) - SH_MAG(6) + SH_MAG(7);
        SK_MZ(3) = 2*magD*q1 + 2*magE*q0 - 2*magN*q3;
        SK_MZ(4) = SH_MAG(8) + SH_MAG(9) - 2*magD*q2;
        SK_MZ(5) = 2*q0*q1 - 2*q2*q3;
        SK_MZ(6) = 2*q0*q2 + 2*q1*q3;
        K_MAG(1,1) = SK_MZ(1)*(P(1,24) + P(1,1)*SH_MAG(2) + P(1,4)*SH_MAG(1) - P(1,2)*SK_MZ(3) + P(1,3)*SK_MZ(4) + P(1,21)*SK_MZ(2) + P(1,19)*SK_MZ(6) - P(1,20)*SK_MZ(5));
        K_MAG(2,1) = SK_MZ(1)*(P(2,24) + P(2,1)*SH_MAG(2) + P(2,4)*SH_MAG(1) - P(2,2)*SK_MZ(3) + P(2,3)*SK_MZ(4) + P(2,21)*SK_MZ(2) + P(2,19)*SK_MZ(6) - P(2,20)*SK_MZ(5));
        K_MAG(3,1) = SK_MZ(1)*(P(3,24) + P(3,1)*SH_MAG(2) + P(3,4)*SH_MAG(1) - P(3,2)*SK_MZ(3) + P(3,3)*SK_MZ(4) + P(3,21)*SK_MZ(2) + P(3,19)*SK_MZ(6) - P(3,20)*SK_MZ(5));
        K_MAG(4,1) = SK_MZ(1)*(P(4,24) + P(4,1)*SH_MAG(2) + P(4,4)*SH_MAG(1) - P(4,2)*SK_MZ(3) + P(4,3)*SK_MZ(4) + P(4,21)*SK_MZ(2) + P(4,19)*SK_MZ(6) - P(4,20)*SK_MZ(5));
        K_MAG(5,1) = SK_MZ(1)*(P(5,24) + P(5,1)*SH_MAG(2) + P(5,4)*SH_MAG(1) - P(5,2)*SK_MZ(3) + P(5,3)*SK_MZ(4) + P(5,21)*SK_MZ(2) + P(5,19)*SK_MZ(6) - P(5,20)*SK_MZ(5));
        K_MAG(6,1) = SK_MZ(1)*(P(6,24) + P(6,1)*SH_MAG(2) + P(6,4)*SH_MAG(1) - P(6,2)*SK_MZ(3) + P(6,3)*SK_MZ(4) + P(6,21)*SK_MZ(2) + P(6,19)*SK_MZ(6) - P(6,20)*SK_MZ(5));
        K_MAG(7,1) = SK_MZ(1)*(P(7,24) + P(7,1)*SH_MAG(2) + P(7,4)*SH_MAG(1) - P(7,2)*SK_MZ(3) + P(7,3)*SK_MZ(4) + P(7,21)*SK_MZ(2) + P(7,19)*SK_MZ(6) - P(7,20)*SK_MZ(5));
        K_MAG(8,1) = SK_MZ(1)*(P(8,24) + P(8,1)*SH_MAG(2) + P(8,4)*SH_MAG(1) - P(8,2)*SK_MZ(3) + P(8,3)*SK_MZ(4) + P(8,21)*SK_MZ(2) + P(8,19)*SK_MZ(6) - P(8,20)*SK_MZ(5));
        K_MAG(9,1) = SK_MZ(1)*(P(9,24) + P(9,1)*SH_MAG(2) + P(9,4)*SH_MAG(1) - P(9,2)*SK_MZ(3) + P(9,3)*SK_MZ(4) + P(9,21)*SK_MZ(2) + P(9,19)*SK_MZ(6) - P(9,20)*SK_MZ(5));
        K_MAG(10,1) = SK_MZ(1)*(P(10,24) + P(10,1)*SH_MAG(2) + P(10,4)*SH_MAG(1) - P(10,2)*SK_MZ(3) + P(10,3)*SK_MZ(4) + P(10,21)*SK_MZ(2) + P(10,19)*SK_MZ(6) - P(10,20)*SK_MZ(5));
        K_MAG(11,1) = SK_MZ(1)*(P(11,24) + P(11,1)*SH_MAG(2) + P(11,4)*SH_MAG(1) - P(11,2)*SK_MZ(3) + P(11,3)*SK_MZ(4) + P(11,21)*SK_MZ(2) + P(11,19)*SK_MZ(6) - P(11,20)*SK_MZ(5));
        K_MAG(12,1) = SK_MZ(1)*(P(12,24) + P(12,1)*SH_MAG(2) + P(12,4)*SH_MAG(1) - P(12,2)*SK_MZ(3) + P(12,3)*SK_MZ(4) + P(12,21)*SK_MZ(2) + P(12,19)*SK_MZ(6) - P(12,20)*SK_MZ(5));
        K_MAG(13,1) = SK_MZ(1)*(P(13,24) + P(13,1)*SH_MAG(2) + P(13,4)*SH_MAG(1) - P(13,2)*SK_MZ(3) + P(13,3)*SK_MZ(4) + P(13,21)*SK_MZ(2) + P(13,19)*SK_MZ(6) - P(13,20)*SK_MZ(5));
        K_MAG(14,1) = SK_MZ(1)*(P(14,24) + P(14,1)*SH_MAG(2) + P(14,4)*SH_MAG(1) - P(14,2)*SK_MZ(3) + P(14,3)*SK_MZ(4) + P(14,21)*SK_MZ(2) + P(14,19)*SK_MZ(6) - P(14,20)*SK_MZ(5));
        K_MAG(15,1) = SK_MZ(1)*(P(15,24) + P(15,1)*SH_MAG(2) + P(15,4)*SH_MAG(1) - P(15,2)*SK_MZ(3) + P(15,3)*SK_MZ(4) + P(15,21)*SK_MZ(2) + P(15,19)*SK_MZ(6) - P(15,20)*SK_MZ(5));
        K_MAG(16,1) = SK_MZ(1)*(P(16,24) + P(16,1)*SH_MAG(2) + P(16,4)*SH_MAG(1) - P(16,2)*SK_MZ(3) + P(16,3)*SK_MZ(4) + P(16,21)*SK_MZ(2) + P(16,19)*SK_MZ(6) - P(16,20)*SK_MZ(5));
        K_MAG(17,1) = SK_MZ(1)*(P(17,24) + P(17,1)*SH_MAG(2) + P(17,4)*SH_MAG(1) - P(17,2)*SK_MZ(3) + P(17,3)*SK_MZ(4) + P(17,21)*SK_MZ(2) + P(17,19)*SK_MZ(6) - P(17,20)*SK_MZ(5));
        K_MAG(18,1) = SK_MZ(1)*(P(18,24) + P(18,1)*SH_MAG(2) + P(18,4)*SH_MAG(1) - P(18,2)*SK_MZ(3) + P(18,3)*SK_MZ(4) + P(18,21)*SK_MZ(2) + P(18,19)*SK_MZ(6) - P(18,20)*SK_MZ(5));
        K_MAG(19,1) = SK_MZ(1)*(P(19,24) + P(19,1)*SH_MAG(2) + P(19,4)*SH_MAG(1) - P(19,2)*SK_MZ(3) + P(19,3)*SK_MZ(4) + P(19,21)*SK_MZ(2) + P(19,19)*SK_MZ(6) - P(19,20)*SK_MZ(5));
        K_MAG(20,1) = SK_MZ(1)*(P(20,24) + P(20,1)*SH_MAG(2) + P(20,4)*SH_MAG(1) - P(20,2)*SK_MZ(3) + P(20,3)*SK_MZ(4) + P(20,21)*SK_MZ(2) + P(20,19)*SK_MZ(6) - P(20,20)*SK_MZ(5));
        K_MAG(21,1) = SK_MZ(1)*(P(21,24) + P(21,1)*SH_MAG(2) + P(21,4)*SH_MAG(1) - P(21,2)*SK_MZ(3) + P(21,3)*SK_MZ(4) + P(21,21)*SK_MZ(2) + P(21,19)*SK_MZ(6) - P(21,20)*SK_MZ(5));
        K_MAG(22,1) = SK_MZ(1)*(P(22,24) + P(22,1)*SH_MAG(2) + P(22,4)*SH_MAG(1) - P(22,2)*SK_MZ(3) + P(22,3)*SK_MZ(4) + P(22,21)*SK_MZ(2) + P(22,19)*SK_MZ(6) - P(22,20)*SK_MZ(5));
        K_MAG(23,1) = SK_MZ(1)*(P(23,24) + P(23,1)*SH_MAG(2) + P(23,4)*SH_MAG(1) - P(23,2)*SK_MZ(3) + P(23,3)*SK_MZ(4) + P(23,21)*SK_MZ(2) + P(23,19)*SK_MZ(6) - P(23,20)*SK_MZ(5));
        K_MAG(24,1) = SK_MZ(1)*(P(24,24) + P(24,1)*SH_MAG(2) + P(24,4)*SH_MAG(1) - P(24,2)*SK_MZ(3) + P(24,3)*SK_MZ(4) + P(24,21)*SK_MZ(2) + P(24,19)*SK_MZ(6) - P(24,20)*SK_MZ(5));
        varInnov(3) = 1/SK_MZ(1);
    end
    % Calculate the measurement innovation
    innovation(obsIndex) = MagPred(obsIndex) - MagData(obsIndex);
    % Check the innovation for consistencey and don't fuse if > 5Sigma
    if ((innovation(obsIndex)^2) / varInnov(obsIndex)) < 25.0
        xk = K_MAG * innovation(obsIndex);
        states = states - xk;
        % normalise the quaternion states
        quatMag = sqrt(states(1)^2 + states(2)^2 + states(3)^2 + states(4)^2);
        if (quatMag > 1e-12)
            states(1:4) = states(1:4) / quatMag;
        end
        % correct the covariance P = (I - K*H)*P
        % take advantage of the empty columns in KH to reduce the
        % number of operations
        for i = 1:24
            for j = 1:4
                KH(i,j) = K_MAG(i,1)*H_MAG(1,j);
            end
            for j = 19:24
                KH(i,j) = K_MAG(i,1)*H_MAG(1,j);
            end
        end
        for i = 1:24
            for j = 1:24
                for k = 1:4
                    KHP(i,j) = KHP(i,j) + KH(i,k)*P(k,j);
                end
                for k = 19:24
                    KHP(i,j) = KHP(i,j) + KH(i,k)*P(k,j);
                end
            end
        end
        P = P - KHP;
    end
    % increment observation index
    obsIndex = obsIndex + 1;
end
% Set output for states and covariance
nextP = P;
nextStates = states;
end

== matlab function NavFilterTestHarness24/LogData/Embedded MATLAB Function ==
  data: eulVar output; states input; quatCov input
%#codegen
function eulVar  = calcEulerVariances(states,quatCov)

eulVar = zeros(1,3);

q0 = states(1);
q1 = states(2);
q2 = states(3);
q3 = states(4);

SJ = zeros(5,1);
SJ(1) = 1/(((2*q0*q3 + 2*q1*q2)/q0^2 + q1^2 - q2^2 - q3^2)^2 + 1);
SJ(2) = 1/(((2*q0*q1 + 2*q2*q3)/q0^2 - q1^2 - q2^2 + q3^2)^2 + 1);
SJ(3) = 1/(1 - (2*q0*q2 - 2*q1*q3)^2)^(1/2);
SJ(4) = 1/q0^2;
SJ(5) = 1/q0^3;

J = zeros(3,4);
J(1,1) = SJ(2)*(2*q1*SJ(4) - 2*SJ(5)*(2*q0*q1 + 2*q2*q3));
J(1,2) = -SJ(2)*(2*q1 - 2/q0);
J(1,3) = -SJ(2)*(2*q2 - 2*q3*SJ(4));
J(1,4) = SJ(2)*(2*q3 + 2*q2*SJ(4));
J(2,1) = 2*q2*SJ(3);
J(2,2) = -2*q3*SJ(3);
J(2,3) = 2*q0*SJ(3);
J(2,4) = -2*q1*SJ(3);
J(3,1) = SJ(1)*(2*q3*SJ(4) - 2*SJ(5)*(2*q0*q3 + 2*q1*q2));
J(3,2) = SJ(1)*(2*q1 + 2*q2*SJ(4));
J(3,3) = -SJ(1)*(2*q2 - 2*q1*SJ(4));
J(3,4) = -SJ(1)*(2*q3 - 2/q0);

% Transform the Euler angle covariances into the equivalent quaternion covariances
eulCov = J*quatCov*transpose(J);

eulVar(1) = eulCov(1,1);
eulVar(2) = eulCov(2,2);
eulVar(3) = eulCov(3,3);


return

== matlab function NavFilterTestHarness24/LogData/Convert GPS Data ==
  data: LatLongDeg input; GndSpd input; CourseDeg input; VelD input; VelNED output; PosNE output; RefLatLongDeg input
%#codegen
function [VelNED,PosNE]   = ConvertGpsData(LatLongDeg,GndSpd,CourseDeg,VelD,RefLatLongDeg)

% Do a conversion from lat,long to local North.Est position relative to a
% reference point using WGS-84 eaerth radius and using a simple spherical
% earth model
% Convert GPS course and speed to North and East velocity components

deg2rad = single(pi/180);
earthRadius = single(6378145);

PosNE = single(zeros(2,1));
VelNED = single(zeros(3,1));
LatLongDelta = (LatLongDeg-RefLatLongDeg) * deg2rad;
PosNE(1) = earthRadius * LatLongDelta(1);
PosNE(2) = earthRadius * cos(RefLatLongDeg(1)*deg2rad) * LatLongDelta(2);
VelNED(1) = GndSpd*cos(CourseDeg*deg2rad);
VelNED(2) = GndSpd*sin(CourseDeg*deg2rad);
VelNED(3) = VelD;

return

== matlab function NavFilterTestHarness24/InertialNavFilter/Recall States5 ==
  data: fuseData output; statesStore input; msecStore input; msecDelay input; statesOut output; states input; time input; newDataArrived input
%#codegen
function [fuseData,statesOut]    = RecallStates5(statesStore,msecStore,msecDelay,states,time,newDataArrived)
persistent statesForFusion;
if isempty(statesForFusion)
    statesForFusion = single(zeros(24,1));
end
bestTimeDelta = int32(msecDelay);
bestStoreIndex = 1;
if newDataArrived
    for storeIndex=1:50
        timeDelta = (int32(time*1000) - int32(msecDelay)) - int32(msecStore(storeIndex));
        if (timeDelta < 0)
            timeDelta = -timeDelta;
        end
        if (timeDelta < bestTimeDelta)
            bestStoreIndex = storeIndex;
            bestTimeDelta = timeDelta;
        end
    end
    if (bestTimeDelta < msecDelay) % only output stored state if time accuracy better than just outputtting current states
        for i=1:24
            statesForFusion(i) = statesStore(i,bestStoreIndex);
        end
    else % otherwise output current state
        for i=1:24
            statesForFusion(i) = states(i);
        end
    end
end
statesOut = statesForFusion;
fuseData = newDataArrived;
end

== matlab function NavFilterTestHarness24/InertialNavFilter/Read Measurements/Convert GPS Data ==
  data: VelNED output; PosNE output; GPS_DataArrived input; RefLatLongDeg input; LatLongDeg input; GndSpd input; CourseDeg input; VelD input
%#codegen
function [VelNED,PosNE]   = ConvertGpsData(GPS_DataArrived,RefLatLongDeg,LatLongDeg,GndSpd,CourseDeg,VelD)

% Do a conversion from lat,long to local North.Est position relative to a
% reference point using WGS-84 eaerth radius and using a simple spherical
% earth model
% Convert GPS course and speed to North and East velocity components

deg2rad = single(pi/180);
earthRadius = single(6378145);

PosNE = single(zeros(2,1));
VelNED = single(zeros(3,1));
LatLongDelta = (LatLongDeg-RefLatLongDeg) * deg2rad;
PosNE(1) = earthRadius * LatLongDelta(1);
PosNE(2) = earthRadius * cos(RefLatLongDeg(1)*deg2rad) * LatLongDelta(2);
VelNED(1) = GndSpd*cos(CourseDeg*deg2rad);
VelNED(2) = GndSpd*sin(CourseDeg*deg2rad);
VelNED(3) = VelD;

return

== matlab function NavFilterTestHarness24/InertialNavFilter/Read Measurements/Calculate Delta Angles & Velocities ==
  data: delAngIMU output; delVelIMU output; angRateIMU input; accelIMU input; dtIMU input
%#codegen
function [delAngIMU,delVelIMU]  = CalcDeltaAngVel(angRateIMU, accelIMU, dtIMU)

persistent prevAngRateIMU;
if isempty(prevAngRateIMU)
    prevAngRateIMU = single([0;0;0]);
end
persistent prevAccelIMU;
if isempty(prevAccelIMU)
    prevAccelIMU = single([0;0;0]);
end

% Apply trapezoidal integration
delAngIMU = 0.5*dtIMU*(angRateIMU + prevAngRateIMU);
delVelIMU = 0.5*dtIMU*(accelIMU   + prevAccelIMU  );

prevAngRateIMU = angRateIMU;
prevAccelIMU   = accelIMU;

end

== matlab function NavFilterTestHarness24/InertialNavFilter/Store States ==
  data: states input; time input; statesStoreOut output; msecStoreOut output
%#codegen
function [statesStoreOut,msecStoreOut]   = StoreStates(states,time)


persistent statesStore;
if isempty(statesStore)
    statesStore = single(zeros(24,50));
end

persistent index;
if isempty(index)
    index = 1;
end

persistent msecStore;
if isempty(msecStore)
    msecStore = uint32(zeros(1,50));
end

if (index > 50)
    index = 1;
end
for i=1:24
    statesStore(i,index) = states(i);
end
msecStore(index) = round(time*1000);
index = index + 1;

statesStoreOut = statesStore;
msecStoreOut =  msecStore;

end

== matlab function NavFilterTestHarness24/InertialNavFilter/Recall States1 ==
  data: fuseData output; statesStore input; msecStore input; msecDelay input; statesOut output; states input; time input; newDataArrived input
%#codegen
function [fuseData,statesOut]    = RecallStates1(statesStore,msecStore,msecDelay,states,time,newDataArrived)
persistent statesForFusion;
if isempty(statesForFusion)
    statesForFusion = single(zeros(24,1));
end
bestTimeDelta = int32(msecDelay);
bestStoreIndex = 1;
if newDataArrived
    for storeIndex=1:50
        timeDelta = (int32(time*1000) - int32(msecDelay)) - int32(msecStore(storeIndex));
        if (timeDelta < 0)
            timeDelta = -timeDelta;
        end
        if (timeDelta < bestTimeDelta)
            bestStoreIndex = storeIndex;
            bestTimeDelta = timeDelta;
        end
    end
    if (bestTimeDelta < msecDelay) % only output stored state if time accuracy better than just outputtting current states
        for i=1:24
            statesForFusion(i) = statesStore(i,bestStoreIndex);
        end
    else % otherwise output current state
        for i=1:24
            statesForFusion(i) = states(i);
        end
    end
end
statesOut = statesForFusion;
fuseData = newDataArrived;
end
